simulink model "Aufgabe_7_simulink"  (Simulink 9.2)
settings: Solver=VariableStepAuto  StartTime=0.0  StopTime=10.0  RelTol=1e-3
settings Model: Creator=danial  LastModifiedBy=danial
settings DataIOCC: LimitDataPoints=off  SaveFormat=Dataset  SignalLoggingSaveFormat=Dataset
settings OptimizationCC: LifeSpan=auto
settings DebuggingCC: UnderspecifiedInitializationDetection=Simplified  MergeDetectMultiDrivingBlocksExec=error  FcnCallInpInsideContextMsg=error  StateNameClashWarn=none  SFUnexpectedBacktrackingDiag=error  SFNoUnconditionalDefaultTransitionDiag=error  SFExecutionAtInitializationDiag=warning
settings HardwareCC: ProdBitPerPointer=64  ProdBitPerSizeT=64  ProdBitPerPtrDiffT=64  ProdLargestAtomicFloat=Float  ProdIntDivRoundTo=Zero  ProdEndianess=LittleEndian  ProdWordSize=64  ProdHWDeviceType=Intel->x86-64 (Windows64)
settings ModelReferenceCC: PropagateSignalLabelsOutOfModel=on
settings SFSimCC: SimUseLocalCustomCode=on
settings RTWCC: RTWUseLocalCustomCode=on
settings CodeAppCC: StateflowObjectComments=off
settings GRTTargetCC: TargetLangStandard=C99 (ISO)  GeneratePreprocessorConditionals=Use local settings  CombineOutputUpdateFcns=on  GRTInterface=off
settings ConfigComp: CovMetricSettings=dwe  CovHtmlReporting=off  CovSaveCumulativeToWorkspaceVar=off  CovSaveSingleToWorkspaceVar=off  CovExternalEMLEnable=on

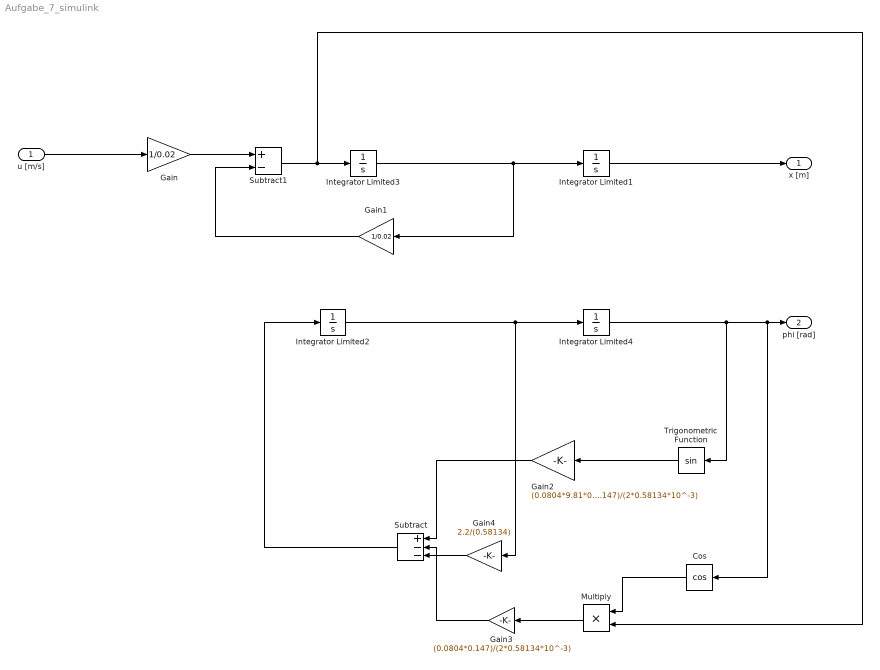
== system Aufgabe_7_simulink ==
  u [m/s] : Inport
  Cos : Trigonometry  Operator=cos
  Gain : Gain  Gain=1/0.02
  Gain1 : Gain  Gain=1/0.02
  Gain2 : Gain  Gain=(0.0804*9.81*0.147)/(2*0.58134*10^-3)
  Gain3 : Gain  Gain=(0.0804*0.147)/(2*0.58134*10^-3)
  Gain4 : Gain  Gain=2.2/(0.58134)
  Integrator Limited1 : Integrator  LimitOutput=on  UpperSaturationLimit=0.25  LowerSaturationLimit=-0.25
  Integrator Limited2 : Integrator  UpperSaturationLimit=1  LowerSaturationLimit=0
  Integrator Limited3 : Integrator  LimitOutput=on  UpperSaturationLimit=0.73  LowerSaturationLimit=-0.73
  Integrator Limited4 : Integrator  InitialCondition=pi  UpperSaturationLimit=1  LowerSaturationLimit=0
  Multiply : Product
  Subtract : Sum  Inputs=+--
  Subtract1 : Sum  Inputs=+-
  Trigonometric Function : Trigonometry
  x [m] : Outport
  phi [rad] : Outport  Port=2
  wires:
  Gain2/1 -> Subtract/1
  Gain3/1 -> Subtract/2
  Gain4/1 -> Subtract/3
  Multiply/1 -> Gain3/1
  Cos/1 -> Multiply/1
  Subtract1/1 -> Multiply/2, Integrator Limited3/1
  Integrator Limited2/1 -> Integrator Limited4/1, Gain4/1
  Trigonometric Function/1 -> Gain2/1
  Integrator Limited1/1 -> x [m]/1
  Subtract/1 -> Integrator Limited2/1
  Integrator Limited3/1 -> Integrator Limited1/1, Gain1/1
  Gain/1 -> Subtract1/1
  Integrator Limited4/1 -> Trigonometric Function/1, Cos/1, phi [rad]/1
  Gain1/1 -> Subtract1/2
  u [m/s]/1 -> Gain/1
